simulink model "videogradfiltraspi"  (R2015a)
settings: Solver=FixedStepDiscrete  StartTime=0.0  StopTime=10.0  RelTol=1e-3
libraries: embdlinuxlib x2
settings Model: SimulationMode=external  CovSFcnEnable=off  ExtModeTrigDuration=100  Creator=Shogo  LastModifiedBy=Shogo
settings OptimizationCC: OptimizeModelRefInitCode=on  LifeSpan=1
settings DebuggingCC: UnderspecifiedInitializationDetection=Classic  MergeDetectMultiDrivingBlocksExec=none
settings HardwareCC: ProdLargestAtomicInteger=Long  ProdLargestAtomicFloat=Double  ProdEndianess=LittleEndian  ProdHWDeviceType=ARM Compatible->ARM Cortex
settings RTWCC: SystemTargetFile=realtime.tlc  GenerateMakefile=off  TemplateMakefile=realtime.tmf  Description=Run on Target Hardware  RTWVerbose=off
settings ERTTargetCC: CombineOutputUpdateFcns=off  ExtMode=on  ExtModeMexArgs='192.168.11.2' 0 17725  ERTSrcFileBannerTemplate=realtime_code_template.cgt  ERTHdrFileBannerTemplate=realtime_code_template.cgt  ERTDataSrcFileTemplate=realtime_code_template.cgt  ERTDataHdrFileTemplate=realtime_code_template.cgt  ERTCustomFileTemplate=realtime_file_process.tlc

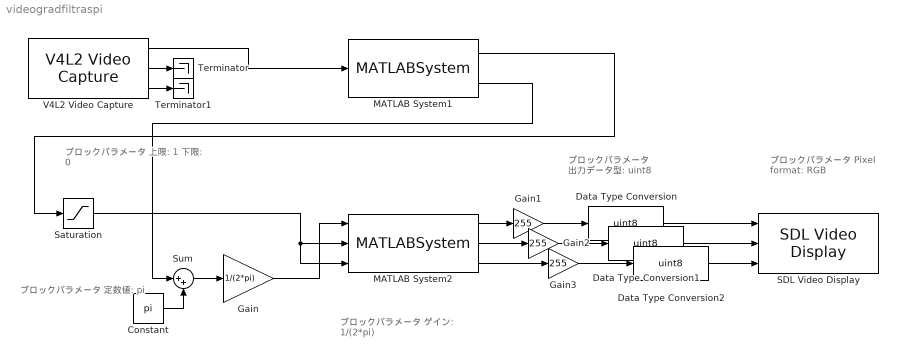
== system videogradfiltraspi ==
  note: ブロックパラメータ
      | Pixel format: RGB
  note: ブロックパラメータ
      | 定数値: pi
  note: ブロックパラメータ
      | 上限: 1
      | 下限: 0
  note: ブロックパラメータ
      | ゲイン: 1/(2*pi)
  note: ブロックパラメータ
      | 出力データ型: uint8
  Constant : Constant  Value=pi
  Data Type Conversion : DataTypeConversion  OutDataTypeStr=uint8
  Data Type Conversion1 : DataTypeConversion  OutDataTypeStr=uint8
  Data Type Conversion2 : DataTypeConversion  OutDataTypeStr=uint8
  Gain : Gain  Gain=1/(2*pi)
  Gain1 : Gain  Gain=255
  Gain2 : Gain  Gain=255
  Gain3 : Gain  Gain=255
  MATLAB System1 : MATLABSystem  System=GradFiltSystem  Kernel=[ 1, 1, 1; 0, 0, 0; -1, -1, -1 ].'  SimulateUsing=Code generation
      mask Type: GradFiltSystem
      mask Display:
      | disp('Grad. Filt.');
      | port_label('input',1,'Gray');
      | port_label('output',1,'Mag.');
      | port_label('output',2,'Ang.');
  MATLAB System2 : MATLABSystem  System=Hsv2RgbSystem  SimulateUsing=Code generation
      mask Type: Hsv2RgbSystem
      mask Display:
      | disp('HSV to RGB');
      | port_label('input',1,'H');
      | port_label('input',2,'S');
      | port_label('input',3,'V');
      | port_label('output',1,'R');
      | port_label('output',2,'G');
      | port_label('output',3,'B');
  SDL Video Display : embdlinuxlib/SDL Video Display  pixelFormat=RGB  pixelOrder=Planar  rowMajor=on  blockPlatform=Raspberry Pi
  Saturation : Saturate  UpperLimit=1  LowerLimit=0
  Sum : Sum  Inputs=|++
  Terminator : Terminator
  Terminator1 : Terminator
  V4L2 Video Capture : embdlinuxlib/V4L2 Video Capture  m_devName='/dev/video0'  roi=[0, 0, 640, 480]  imSizeSelection=320x240  imSize=[640, 480]  pixelFormat=YCbCr 4:2:2  pixelOrder=Planar  sampleTime=1/5  simOutput=Colorbars  blockPlatform=Raspberry Pi
  wires:
  V4L2 Video Capture/1 -> MATLAB System1/1
  MATLAB System2/1 -> Gain1/1
  MATLAB System2/2 -> Gain2/1
  MATLAB System2/3 -> Gain3/1
  MATLAB System1/1 -> Saturation/1
  Saturation/1 -> MATLAB System2/2, MATLAB System2/3
  Gain/1 -> MATLAB System2/1
  MATLAB System1/2 -> Sum/1
  Sum/1 -> Gain/1
  Constant/1 -> Sum/2
  V4L2 Video Capture/2 -> Terminator/1
  V4L2 Video Capture/3 -> Terminator1/1
  Gain1/1 -> Data Type Conversion/1
  Gain2/1 -> Data Type Conversion1/1
  Gain3/1 -> Data Type Conversion2/1
  Data Type Conversion/1 -> SDL Video Display/1
  Data Type Conversion1/1 -> SDL Video Display/2
  Data Type Conversion2/1 -> SDL Video Display/3
